simulink model "Vehicle14DOFSystemRack"  (R2024a)
settings: Solver=ode4  StartTime=0.0  StopTime=100  FixedStep=0.001  RelTol=1e-3
values from neighbouring files (symbols this model uses):
  EnvGrvty = 9.81    [Par.m]
  PlntBattChrgMax = 4.493    [Par.m]
  PlntBattNumCellSer = 96    [Par.m]
  PlntBattOpenCirctVolt = [3.17242 3.17242 3.17242 3.17242 3.17242 3.17242 3.17242;3.18272 3.18272 3.18272 3.18272 3.18272 3.18272 3.18272;3.19302 3.19302 3.19302 3.19302 3.19302 3.19302 3.19302;3.20331 3.20331 3.20331 3.20331 3.20331 3.20331 3.20331;3.21361 3.21361 3.21361 3.21361 3.21361 3.21361 3.21361;3.22391 3.22391 3.22391 3.22391 3.22391 3.22391 3.22391;3.23421 3.23421 3.23421 3.23421 3.23421 3.23421 3.23421;3.24451 ...(+5187 chars)    [Par.m]
  PlntBattSocInit = 0.6    [Par.m]
  PlntBattTempBpt = [-40 -30 -20 0 23 45 60]    [Par.m]
  PlntBattTempInitDegC = 25    [Par.m]
  PlntBattVoltSocBpt = [0 0.01 0.02 0.03 0.04 0.05 0.06 0.07 0.08 0.09 0.1 0.11 0.12 0.13 0.14 0.15 0.16 0.17 0.18 0.19 0.2 0.21 0.22 0.23 0.24 0.25 0.26 0.27 0.28 0.29 0.3 0.31 0.32 0.33 0.34 0.35 0.36 0.37 0.38 0.39 0.4 0.41 0.42 0.43 0.44 0.45 0.46 0.47 0.48 0.49 0.5 0.51 0.52 0.53 0.54 0.55 0.56 0.57 0.58 0.59 0.6 0.61 0.62 0.63 0.64 0.65 0.66 0.67 0.68 0.69 0.7 0.71 0.72 0.73 0.74 0.75 0.76 0.77 0.78 0.79 0.8 0.81  ...(+91 chars)    [Par.m]
  PlntDCDCVoltInit = 650    [Par.m]
  PlntDriveshftDamp = 100    [Par.m]
  PlntDriveshftStiff = 500    [Par.m]
  PlntEM1RotDamp = 0.001    [Par.m]
  PlntEM1RotInertia = 0.01    [Par.m]
  PlntEM2RotDamp = 0.001    [Par.m]
  PlntEM2RotInertia = 0.01    [Par.m]
  PlntEM3RotDamp = 0.001    [Par.m]
  PlntEM3RotInertia = 0.01    [Par.m]
  PlntEM4RotDamp = 0.001    [Par.m]
  PlntEM4RotInertia = 0.01    [Par.m]
  PlntEMWhlGearRatioFL = 11.04    [Par.m]
  PlntEMWhlGearRatioFR = 11.04    [Par.m]
  PlntEMWhlGearRatioRL = 11.04    [Par.m]
  PlntEMWhlGearRatioRR = 11.04    [Par.m]
  PlntSteerGearRatio = 52.025    [Par.m]
  PlntVehCGHgtAxl = 0.375    [Par.m]
  PlntVehDstCGFrntAxl = 1.61    [Par.m]
  PlntVehDstCGRearAxl = 1.39    [Par.m]
  PlntVehFrntUnsprgMass = 100    [Par.m]
  PlntVehInitLatPos = 0    [Par.m]
  PlntVehInitLatVel = 0    [Par.m]
  PlntVehInitLongPos = 0    [Par.m]
  PlntVehInitLongVel = 0    [Par.m]
  PlntVehInitPitchAng = 0    [Par.m]
  PlntVehInitPitchRate = 0    [Par.m]
  PlntVehInitRollAng = 0    [Par.m]
  PlntVehInitRollRate = 0    [Par.m]
  PlntVehInitVertPos = 0    [Par.m]
  PlntVehInitVertVel = 0    [Par.m]
  PlntVehInitYawAng = 0    [Par.m]
  PlntVehInitYawRate = 0    [Par.m]
  PlntVehMass = 2497    [Par.m]
  PlntVehPitchMomentInertia = 1922.7    [Par.m]
  PlntVehRearUnsprgMass = 100    [Par.m]
  PlntVehRollMomentInertia = 432.33333333333331    (= 432.333333333)    [Par.m]
  PlntVehTrckWdth = [1.685,1.685]    [Par.m]
  PlntVehYawMomentInertia = 2066    [Par.m]
  PlntWhlNumFrnt = 2    [Par.m]
  PlntWhlNumRear = 2    [Par.m]
  PlntWhlPrsFrnt = 220000    [Par.m]
  PlntWhlPrsRear = 220000    [Par.m]
libraries: autolibsharedcoupling x12, autolibsharedcommon x12, autolibutils x10, autolibmappedmotor x4, autolibcoupling x4, matrix_library x4, vehdynlibsteering x4, vehdynlibsuspension x2, vehdynlibtire x2, vehdynlibtirecommon x2, shared6dof x2, autolibdatasheetbattery x1
(part 6 of 7)

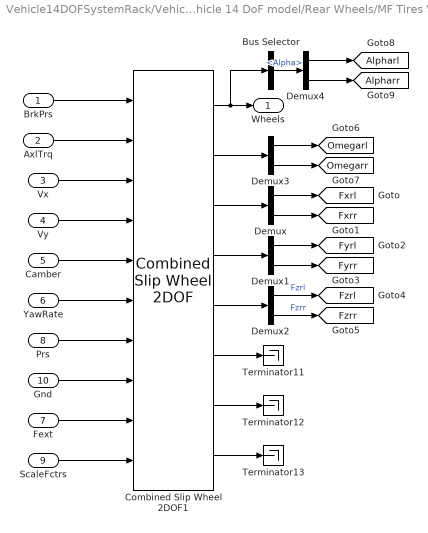
== system Vehicle14DOFSystemRack/Vehicle 14 DoF model/Vehicle 14 DoF model/Rear Wheels/MF Tires Vector ==
  BrkPrs : Inport
  AxlTrq : Inport  Port=2
  Vx : Inport  Port=3
  Vy : Inport  Port=4
  Camber : Inport  Port=5
  YawRate : Inport  Port=6
  Fext : Inport  Port=7
  Prs : Inport  Port=8  Unit=Pa
  ScaleFctrs : Inport  Port=9  Unit=1
  Gnd : Inport  Port=10
  Bus Selector : BusSelector  OutputSignals=Alpha
  Combined Slip Wheel 2DOF1 : vehdynlibtire/Combined Slip Wheel 2DOF  tireType=SUV 265/50R20  BrakeType=Disc  vertType=Magic Formula  plySteer=off  turnslip=on  mu_static=.3  mu_kinetic=.2  disk_abore=.05  Rm=.177  num_pads=2  drum_abore=0.0508  drum_a=0.123  drum_c=0.212  drum_r=0.15  drum_theta1=0  drum_theta2=126  brake_p_bpt=[1 11.4736842105263 21.9473684210526 32.4210526315789 42.8947368421053 53.3684210526316 63.8421052631579 74.3157894736842 84.7894736842105 95.2631578947368 105.736842105263 116.210526315789 126.684210526316 137.157894736842 147.631578947368 158.105263157895 168.578947368421 179.052631578947 189.526315789474 200]  brake_n_bpt=[0 52.6315789473684 105.263157894737 157.894736842105 210.526315789474 263.157894736842 315.789473684211 368.421052631579 421.052631578947 473.684210526316 526.315789473684 578.947368421053 631.578947368421 684.210526315789 736.842105263158 789.473684210526 842.105263157895 894.736842105263 947.368421052632 1000]  f_brake_t=[43.4900602404453 42.5056030554862 41.5350898940194 40.5780454442085 39.6340111501808 38.7025443887544 37.7832176914519 36.8756180088306 35.9793460143796 35.0940154454303 34.2192524787115 33.3546951383474 32.4999927342521 31.6548053290159 30.8188032315107 29.991666515561 29.1730845621415 28.362755623661 27.5603864089927 26.765691687993;498.991217495636 487.695866636631 476.560505099801 465.579679307235 454.748127933653 444.060772460445 433.51270824929 423.099196101319 412.81565427025 402.657650900201 392.620896861006 382.701238955775 372.894653477208 363.197240090814 353.605216024701 344.114910546964 334.722759712992 325.425301366216 316.219170376863 307.10109410434;954.492374750826 932.886130217776 911.585920305583 890.581313170261 869.862244717126 849.419000532136 829.242198807128 809.322774193808 789.651962526121 770.221286354971 751.0225412433 732.047782773203 713.289314220164 694.739674852612 676.391628817892 658.238154578366 640.272434863842 622.48784710877 604.877954344734 587.436496520688;1409.99353200602 1378.07639379892 1346.61133551136 1315.58294703329 1284.9763615006 1254.77722860383 1224.97168936497 1195.5463522863 1166.48827078199 1137.78492180974 1109.42418562559 1081.39432659063 1053.68397496312 1026.28210961441 999.178041611083 972.361398609768 945.822110014692 919.550392851325 893.536738312604 867.771898937035;1865.49468926121 1823.26665738007 1781.63675071715 1740.58458089631 1700.09047828407 1660.13545667552 1620.7011799228 1581.76993037878 1543.32457903786 1505.34855726451 1467.82583000789 1430.74087040806 1394.07863570608 1357.82454437621 1321.96445440427 1286.48464264117 1251.37178516554 1216.61293859388 1182.19552228048 1148.10730135338;2320.9958465164 2268.45692096121 2216.66216592293 2165.58621475934 2115.20459506754 2065.49368474721 2016.43067048064 1967.99350847127 1920.16088729373 1872.91219271928 1826.22747439018 1780.08741422549 1734.47329644903 1689.36697913801 1644.75086719747 1600.60788667257 1556.92146031639 1513.67548433643 1470.85430624835 1428.44270376973;2776.49700377159 2713.64718454235 2651.68758112871 2590.58784862237 2530.31871185102 2470.8519128189 2412.16016103848 2354.21708656376 2296.9971955496 2240.47582817405 2184.62911877248 2129.43395804292 2074.86795719199 2020.9094138998 1967.53727999066 1914.73113070398 1862.47113546724 1810.73803007899 1759.51309021622 1708.77810618608;3231.99816102678 3158.8374481235 3086.71299633449 3015.58948248539 2945.43282863449 2876.21014089059 2807.88965159632 2740.44066465625 2673.83350380547 2608.03946362882 2543.03076315477 2478.78050186034 2415.26261793494 2352.4518486616 2290.32369278385 2228.85437473538 2168.02081061809 2107.80057582154 2048.17187418409 1989.11350860242;3687.49931828197 3604.02771170464 3521.73841154027 3440.59111634842 3360.54694541796 3281.56836896228 3203.61914215416 3126.66424274874 3050.66981206134 2975.60309908359 2901.43240753707 2828.12704567777 2755.6572786779 2683.9942834234 2613.11010557704 2542.97761876678 2473.57048576894 2404.8631215641 2336.83065815196 2269.44891101877;4143.00047553716 4049.21797528579 3956.76382674606 3865.59275021144 3775.66106220143 3686.92659703397 3599.34863271199 3512.88782084123 3427.50612031721 3343.16673453836 3259.83405191936 3177.4735894952 3096.05193942085 3015.5367181852 2935.89651837023 2857.10086279818 2779.12016091979 2701.92566730665 2625.48944211983 2549.78431343512;4598.50163279235 4494.40823886693 4391.78924195184 4290.59438407447 4190.77517898491 4092.28482510566 3995.07812326983 3899.11139893372 3804.34242857308 3710.73036999313 3618.23569630166 3526.82013331263 3436.44660016381 3347.079152947 3258.68293116342 3171.22410682959 3084.66983607064 2998.98821304921 2914.1482260877 2830.11971585147;5054.00279004754 4939.59850244808 4826.81465715762 4715.59601793749 4605.88929576838 4497.64305317735 4390.80761382767 4285.3349770262 4181.17873682896 4078.2940054479 3976.63734068395 3876.16667713006 3776.84126090677 3678.62158770879 3581.46934395661 3485.34735086099 ...(+2764 chars)]  tireParamSet=vdynPassCar.mat  PRESMAX=1000000  PRESMIN=10000  FZMAX=12400  FZMIN=100  VXLOW=0.1  KPUMAX=1.5  KPUMIN=-1.5  ALPMAX=1.5  ALPMIN=-1.5  CAMMAX=0.17453  CAMMIN=-0.17453  LONGVL=16.7  FxRelFreqLwrLim=200*pi  FyRelFreqLwrLim=200*pi  MyRelFreqLwrLim=100*pi  omegao=20/0.3869  br=1e-3  UNLOADED_RADIUS=0.3869  NOMPRES=269000  FNOMIN=6200  WIDTH=0.265  RIM_RADIUS=0.254  MASS=16.15  IYY=2.081  GRAVITY=-9.81  zo=0  zdoto=0  BREFF=8.25094594147963  DREFF=0.260468730454265  FREFF=0.0735298544471851  Q_RE0=1.00866439868088  Q_V1=0.000760413786224011  Q_V2=0.0463384792019201  Q_FZ1=0  Q_FZ2=15.6870832810226  Q_FZ3=0  Q_FCX=0.138643970247602  Q_FCY=0.10843499565426  Q_FCY2=-0.465763352339538  PFZ1=0.69958166705601  VERTICAL_STIFFNESS=207885.061134007  VERTICAL_DAMPING=500  BOTTOM_OFFST=.01  BOTTOM_STIFF=2e6  LONGITUDINAL_STIFFNESS=388714.175879854  LATERAL_STIFFNESS=157087.404633332  PCFX1=0.18539229191199  PCFX2=0  PCFX3=0  PCFY1=0.163183345037677  PCFY2=0  PCFY3=0.249094918231954  Q_RA1=0.675942571700787  Q_RA2=0.73800463546164  Q_RB1=1.04487486456705  Q_RB2=-1.191763806629  PCX1=1.58523057950359  PDX1=1.0239116238178  PDX2=-0.0842405110022724  PDX3=0  PEX1=0.110312777158455  PEX2=0.313468516038146  PEX3=0  PEX4=0.0016060905760045  PKX1=21.3872544684023  PKX2=14.0006541873175  PKX3=-0.405326109653452  PHX1=0.000212599305364818  PHX2=0.00115950515263055  PVX1=1.59236164471432e-05  PVX2=0.000104321112127671  PPX1=-0.349461321276586  PPX2=0.387840040616429  PPX3=-0.0969947336569324  PPX4=0.0632271859795801  RBX1=12.7633329850276  RBX2=9.5787123658471  RBX3=0  RCX1=1.02796280922059  REX1=-0.45202516851367  REX2=-0.47304886171176  RHX1=0.000233272373115809  QSX1=-0.00788307788961443  QSX2=0.954629515459396  QSX3=0.0155855777667025  QSX4=0.125904607142414  QSX5=1.01110069703963  QSX6=20.1938577118433  QSX7=0.310818120717083  QSX8=-0.0430823751139655  QSX9=0.636494404888216  QSX10=0.142438060591663  QSX11=0.346766530036373  QSX12=0  QSX13=0  QSX14=0  PPMX1=0  PCY1=1.34299950037631  PDY1=0.878267729082195  PDY2=-0.0644597923147385  PDY3=0  PEY1=-0.809776534470972  PEY2=-0.600180598867198  PEY3=0.0991732552633487  PEY4=-6.5577974035573  PEY5=0  PKY1=-15.5714726518315  PKY2=1.73126522291751  PKY3=0.365349873517229  PKY4=1.98176755955416  PKY5=0  PKY6=-0.884005199550313  PKY7=-0.237259727611847  PHY1=-0.00183370557235628  PHY2=0.00346401302716671  PVY1=-0.00675427560163264  PVY2=0.036379218103843  PVY3=-0.163543984089166  PVY4=-0.491003349625726  PPY1=-0.62059646553185  PPY2=-0.0647824842338686  PPY3=-0.164648843290686  PPY4=0.283193909060098  PPY5=0  RBY1=10.7588809173639  RBY2=7.70420065295029  RBY3=3.40283755070691e-06  RBY4=0  RCY1=1.06691874059059  REY1=0.308244924574305  REY2=7.48775032604508e-06  RHY1=0.0118479204960415  RHY2=7.63650177161071e-06  RVY1=0.0560024425050078  RVY2=7.48487127056197e-06  RVY3=0  RVY4=98.4047026517149  RVY5=2.02759273900054  RVY6=15.7623064923347  QSY1=0.00699077564863536  QSY2=0  QSY3=0.00153535478298811  QSY4=8.55710322455322e-05  QSY5=0  QSY6=0  QSY7=0.89443879773793  QSY8=-0.403227641260894  QBZ1=11.666656027484  QBZ2=-1.30355438574485  QBZ3=0  QBZ4=0.177918305399071  QBZ5=-0.162481135068033  QBZ6=0  QBZ9=30.1445534682089  QBZ10=0  QCZ1=1.29026978207574  QDZ1=0.0886972644991399  QDZ2=-0.0058634820161856  QDZ3=0.3805597481383  QDZ4=0  QDZ6=0.00160914918118959  QDZ7=-0.00211036330862154  QDZ8=-0.13921904912557  QDZ9=0.00816585550028243  QDZ10=0  QDZ11=0  QEZ1=-2.19802254534746  QEZ2=1.01850535789165  QEZ3=0  QEZ4=0.278379679112054  QEZ5=-0.548414722765386  QHZ1=0.00148361198869669  QHZ2=0.00202017567585904  QHZ3=0.240316641332066  QHZ4=-0.210114035738085  PPZ1=-0.443927982388615  PPZ2=0  SSZ1=0.00914999585397887  SSZ2=0.0389830656052735  SSZ3=0  SSZ4=0  PDXP1=0.396718274678791  PDXP2=0  PDXP3=0  PKYP1=1.00587060633573  PDYP1=0.40483048923438  PDYP2=0  PDYP3=0  PDYP4=0  PHYP1=0.992731942067188  PHYP2=0.150352945499914  PHYP3=0  PHYP4=-3.98988682633674  PECP1=0.502379254513503  PECP2=0  QDTP1=10.0178654287947  QCRP1=0.200627747200702  QCRP2=0.0995735881599772  QBRP1=0.0997107127960717  QDRP1=1.01432910167423  QDRP2=0  aMode=2
  Demux{,1..4} (5 alike) : Demux  Outputs=2
  Terminator11 : Terminator
  Terminator12 : Terminator
  Terminator13 : Terminator
  Wheels : Outport  VectorParamsAs1DForOutWhenUnconnected=off
  tag scope: Alpharl=global, Alpharr=global, Fxrl=global, Fxrr=global, Fyrl=global, Fyrr=global, Fzrl=global, Fzrr=global, Omegarl=global, Omegarr=global
  wires:
  Vy/1 -> Combined Slip Wheel 2DOF1/4
  Combined Slip Wheel 2DOF1/8 -> Terminator13/1
  Combined Slip Wheel 2DOF1/7 -> Terminator12/1
  Combined Slip Wheel 2DOF1/6 -> Terminator11/1
  Fext/1 -> Combined Slip Wheel 2DOF1/9
  Gnd/1 -> Combined Slip Wheel 2DOF1/8
  Prs/1 -> Combined Slip Wheel 2DOF1/7
  YawRate/1 -> Combined Slip Wheel 2DOF1/6
  Camber/1 -> Combined Slip Wheel 2DOF1/5
  Vx/1 -> Combined Slip Wheel 2DOF1/3
  AxlTrq/1 -> Combined Slip Wheel 2DOF1/2
  BrkPrs/1 -> Combined Slip Wheel 2DOF1/1
  ScaleFctrs/1 -> Combined Slip Wheel 2DOF1/10
  Demux3/2 -> [Omegarr]
  Demux3/1 -> [Omegarl]
  Demux1/2 -> [Fyrr]
  Demux1/1 -> [Fyrl]
  Combined Slip Wheel 2DOF1/2 -> Demux3/1
  Combined Slip Wheel 2DOF1/4 -> Demux1/1
  Combined Slip Wheel 2DOF1/5 -> Demux2/1
  Demux2/2 -> [Fzrr]  "Fzrr"
  Combined Slip Wheel 2DOF1/3 -> Demux/1
  Demux2/1 -> [Fzrl]  "Fzrl"
  Demux/2 -> [Fxrr]
  Demux/1 -> [Fxrl]
  Combined Slip Wheel 2DOF1/1 -> Bus Selector/1, Wheels/1
  Demux4/1 -> [Alpharl]
  Bus Selector/1 -> Demux4/1  "<Alpha>"
  Demux4/2 -> [Alpharr]

== system Vehicle14DOFSystemRack/Vehicle 14 DoF model/Vehicle 14 DoF model/Rear Wheels/Rear Friction ==
  u : Inport
  Selector1 : Selector  InputPortWidth=4  IndexOptions=Index vector (dialog)  Indices=[3 4]  OutputSizes=1
  y : Outport
  wires:
  Selector1/1 -> y/1
  u/1 -> Selector1/1

== system Vehicle14DOFSystemRack/Vehicle 14 DoF model/Vehicle 14 DoF model/Rear Wheels/Rear Ground ==
  u : Inport
  Selector1 : Selector  InputPortWidth=4  IndexOptions=Index vector (dialog)  Indices=[3 4]  OutputSizes=1
  y : Outport
  wires:
  u/1 -> Selector1/1
  Selector1/1 -> y/1

== system Vehicle14DOFSystemRack/Vehicle 14 DoF model/Vehicle 14 DoF model/Rear Wheels/Subsystem ==
  lamda_mu_x : Inport
  lamda_mu_y : Inport  Port=2
  Rear Pressure : vehdynlibtirecommon/Constant  const=PlntWhlPrsRear  numWheels=PlntWhlNumRear
  scale factors with friction : Subsystem  mask{numWheels=PlntWhlNumRear}
      mask prompts: numWheels "Number of wheels"
  Prs : Outport
  ScaleFctrs : Outport  Port=2
  wires:
  lamda_mu_y/1 -> scale factors with friction/2(lamda_mu_y)
  scale factors with friction/1(lambdas) -> ScaleFctrs/1
  lamda_mu_x/1 -> scale factors with friction/1(lamda_mu_x)
  Rear Pressure/1 -> Prs/1

== system Vehicle14DOFSystemRack/Vehicle 14 DoF model/Vehicle 14 DoF model/Transfer Case/DriveshftTrq Routing ==
  TrnsfrCaseFrntTrq : Inport
  DriveshftTrq : Inport  Port=2
  "TrnsfrCaseRearTrq " : Inport  Port=3
  Constant : Constant  Value=0  SampleTime=-1
  FrntDiffrntlTrq : Outport
  TrnsfrCaseTrq : Outport  Port=2
  RearDiffrntlTrq : Outport  Port=3
  wires:
  DriveshftTrq/1 -> FrntDiffrntlTrq/1, RearDiffrntlTrq/1
  Constant/1 -> TrnsfrCaseTrq/1

== system Vehicle14DOFSystemRack/Vehicle 14 DoF model/Vehicle 14 DoF model/Transfer Case/Subsystem ==
  TrqSplitRatio : Inport
  SpdLock : Inport  Port=2
  FrntDiffrntlSpd : Inport  Port=3
  DriveshftTrq : Inport  Port=4
  RearDiffrntlSpd : Inport  Port=5
  Constant : Constant  Value=0  SampleTime=-1
  Constant1 : Constant  Value=0  SampleTime=-1
  Constant2 : Constant  Value=0  SampleTime=-1
  DriveshftSpd : Outport
  FrntDiffrntlTrq : Outport  Port=2
  RearDiffrntlTrq : Outport  Port=3
  wires:
  Constant2/1 -> RearDiffrntlTrq/1
  Constant1/1 -> FrntDiffrntlTrq/1
  Constant/1 -> DriveshftSpd/1

== system Vehicle14DOFSystemRack/Vehicle 14 DoF model/Vehicle 14 DoF model/Transmission/BEV4 ==
  EMTrq : Inport
  DriveshftSpd : Inport  Port=2
  Bus Creator : BusCreator  Inputs=4
  Bus Creator1 : BusCreator  Inputs=4
  Bus Selector : BusSelector  OutputSignals=FrntDriveshftSpd.DriveshftSpd1
  Bus Selector1 : BusSelector  OutputSignals=FrntDriveshftSpd.DriveshftSpd2
  Bus Selector2 : BusSelector  OutputSignals=RearDriveshftSpd.DriveshftSpd3
  Bus Selector3 : BusSelector  OutputSignals=RearDriveshftSpd.DriveshftSpd4
  Bus Selector4 : BusSelector  OutputSignals=EMTrq1
  Bus Selector5 : BusSelector  OutputSignals=EMTrq2
  Bus Selector6 : BusSelector  OutputSignals=EMTrq3
  Bus Selector7 : BusSelector  OutputSignals=EMTrq4
  Driveshaft Compliance{,1..3} (4 alike) : autolibsharedcoupling/Torsional Compliance  port_config=Simulink  extInfo=off  k=PlntDriveshftStiff  b=PlntDriveshftDamp  theta_o=PlntDriveshftInitDeflect  domega_o=PlntDriveshftInitVel  omega_c=PlntDriveshftDampCutoffFreq  blkID=0  aMode=1
  Rotational Inertia : autolibsharedcoupling/Rotational Inertia  port_config=Simulink  extInfo=off  externJ=off  J=PlntEM1RotInertia  b=PlntEM1RotDamp  omega_o=PlntEM1RotInitSpd  blkID=0  aMode=1
      settings: LibrarySourceBlock=autolibcoupling/Rotational Inertia
  Rotational Inertia1 : autolibsharedcoupling/Rotational Inertia  port_config=Simulink  extInfo=off  externJ=off  J=PlntEM2RotInertia  b=PlntEM2RotDamp  omega_o=PlntEM2RotInitSpd  blkID=0  aMode=1
      settings: LibrarySourceBlock=autolibcoupling/Rotational Inertia
  Rotational Inertia2 : autolibsharedcoupling/Rotational Inertia  port_config=Simulink  extInfo=off  externJ=off  J=PlntEM3RotInertia  b=PlntEM3RotDamp  omega_o=PlntEM3RotInitSpd  blkID=0  aMode=1
      settings: LibrarySourceBlock=autolibcoupling/Rotational Inertia
  Rotational Inertia3 : autolibsharedcoupling/Rotational Inertia  port_config=Simulink  extInfo=off  externJ=off  J=PlntEM4RotInertia  b=PlntEM4RotDamp  omega_o=PlntEM4RotInitSpd  blkID=0  aMode=1
      settings: LibrarySourceBlock=autolibcoupling/Rotational Inertia
  EMSpd : Outport  VectorParamsAs1DForOutWhenUnconnected=off  BusOutputAsStruct=on
  DriveshftTrq : Outport  Port=2  VectorParamsAs1DForOutWhenUnconnected=off
  wires:
  Bus Selector2/1 -> Driveshaft Compliance2/2  "<DriveshftSpd3>"
  Rotational Inertia1/1 -> Bus Creator1/2, Driveshaft Compliance1/1  "EMSpd2"
  Bus Creator/1 -> DriveshftTrq/1
  Bus Selector4/1 -> Rotational Inertia/1  "<EMTrq1>"
  EMTrq/1 -> Bus Selector4/1, Bus Selector5/1, Bus Selector7/1, Bus Selector6/1
  Bus Selector3/1 -> Driveshaft Compliance3/2  "<DriveshftSpd4>"
  Rotational Inertia/1 -> Bus Creator1/1, Driveshaft Compliance/1  "EMSpd1"
  Bus Selector/1 -> Driveshaft Compliance/2  "<DriveshftSpd1>"
  Bus Selector7/1 -> Rotational Inertia3/1  "<EMTrq4>"
  Driveshaft Compliance3/1 -> Rotational Inertia3/2
  Driveshaft Compliance/1 -> Rotational Inertia/2
  Bus Selector5/1 -> Rotational Inertia1/1  "<EMTrq2>"
  Driveshaft Compliance1/1 -> Rotational Inertia1/2
  DriveshftSpd/1 -> Bus Selector/1, Bus Selector1/1, Bus Selector3/1, Bus Selector2/1
  Driveshaft Compliance3/2 -> Bus Creator/4  "DriveshftTrq4"
  Bus Creator1/1 -> EMSpd/1
  Driveshaft Compliance2/1 -> Rotational Inertia2/2
  Rotational Inertia2/1 -> Bus Creator1/3, Driveshaft Compliance2/1  "EMSpd3"
  Bus Selector1/1 -> Driveshaft Compliance1/2  "<DriveshftSpd2>"
  Rotational Inertia3/1 -> Bus Creator1/4, Driveshaft Compliance3/1  "EMSpd4"
  Bus Selector6/1 -> Rotational Inertia2/1  "<EMTrq3>"
  Driveshaft Compliance2/2 -> Bus Creator/3  "DriveshftTrq3"
  Driveshaft Compliance1/2 -> Bus Creator/2  "DriveshftTrq2"
  Driveshaft Compliance/2 -> Bus Creator/1  "DriveshftTrq1"

== system Vehicle14DOFSystemRack/Vehicle 14 DoF model/Vehicle 14 DoF model/Vehicle Body/Subsystem ==
  Veh : Inport
  Bus Creator : BusCreator  Inputs=2
  Bus Selector : BusSelector  OutputSignals=BdyFrm.Cg.Acc.ax,BdyFrm.Cg.Acc.ay,BdyFrm.Cg.Acc.az  OutputAsBus=on
  Bus Selector1 : BusSelector  OutputSignals=BdyFrm.Cg.AngVel.p,BdyFrm.Cg.AngVel.q,BdyFrm.Cg.AngVel.r  OutputAsBus=on
  Bus Selector2 : BusSelector  OutputSignals=BdyFrm.Cg.AngAcc.pdot,BdyFrm.Cg.AngAcc.qdot,BdyFrm.Cg.AngAcc.rdot  OutputAsBus=on
  Bus to Vector : BusToVector
  Bus to Vector1 : BusToVector
  Bus to Vector2 : BusToVector
  Constant : Constant  Value=[0,0,0]
  Constant1 : Constant  Value=[0,0,9.81]
  Three-axis Inertial Measurement Unit : vehdynlibsens/Three-axis Inertial Measurement Unit  units=Metric (MKS)  imu=[0 0 0]  i_Ts=0  dtype_a=off  w_a=190  z_a=0.707  a_sf_cc=[1 0 0; 0 1 0; 0 0 1]  a_bias=[0 0 0]  a_sat="[-inf  -inf  -inf  inf inf inf]"  dtype_g=off  w_g=190  z_g=0.707  g_sf_cc=[1 0 0; 0 1 0; 0 0 1]  g_bias=[0 0 0]  g_sens=[0 0 0]  g_sat="[-inf  -inf  -inf  inf inf inf]"  i_rand=on  i_seeds=[23093 23094 23095 23096 23097 23098]  i_pow=[0.001 0.001 0.001 0.0001 0.0001 0.0001]  aMode=2
  Unit Conversion : UnitConversion
  IMU : Outport
  wires:
  Three-axis Inertial Measurement Unit/2 -> Bus Creator/2  "Omega"
  Veh/1 -> Bus Selector2/1, Bus Selector1/1, Bus Selector/1
  Constant1/1 -> Three-axis Inertial Measurement Unit/5
  Bus to Vector1/1 -> Three-axis Inertial Measurement Unit/2
  Bus to Vector/1 -> Unit Conversion/1
  Bus Selector1/1 -> Bus to Vector1/1
  Constant/1 -> Three-axis Inertial Measurement Unit/4
  Three-axis Inertial Measurement Unit/1 -> Bus Creator/1  "Ameans"
  Bus Selector2/1 -> Bus to Vector2/1
  Unit Conversion/1 -> Three-axis Inertial Measurement Unit/1
  Bus to Vector2/1 -> Three-axis Inertial Measurement Unit/3
  Bus Selector/1 -> Bus to Vector/1
  Bus Creator/1 -> IMU/1

== system Vehicle14DOFSystemRack/Vehicle 14 DoF model/Vehicle 14 DoF model/Vehicle Body/Vehicle 6DOF ==
  Suspension : Inport
  Constant{1..4} (4 alike) : Constant  Value=[0;0;0]  SampleTime=-1
  Suspension to Chasiss Transforms : Subsystem
  Terminator{,1..5} (6 alike) : Terminator
  Vehicle Body 6DOF : vehdynlibeom/Vehicle Body 6DOF  extPos=on  extVel=on  extEuler=on  extRotRate=on  htchFMode=on  htchMMode=on  m=PlntVehMass  a=PlntVehDstCGFrntAxl  b=PlntVehDstCGRearAxl  d=0  h=PlntVehCGHgtAxl  dh=PlntVehHtchDst  hl=0  hh=PlntVehHtchHgtAxl  Xe_o=[PlntVehInitLongPos, PlntVehInitLatPos, PlntVehInitVertPos]  xbdot_o=[PlntVehInitLongVel+20, PlntVehInitLatVel, PlntVehInitVertVel]  eul_o=[PlntVehInitRollAng, PlntVehInitPitchAng, PlntVehInitYawAng]  p_o=[PlntVehInitRollRate, PlntVehInitPitchRate, PlntVehInitYawRate]  Iveh=[PlntVehRollMomentInertia 0 0; 0 PlntVehPitchMomentInertia 0; 0 0 PlntVehYawMomentInertia]  w=PlntVehTrckWdth  z1m=0  z1R=[-.25,.125,.15]  z1I=[1.4,-.2,.1;-.2,1.4,.1;.1,.1,2.25].*0  z2m=0  z2R=[1.4,0,.8]  z2I=[1.4,-.2,.1;-.2,1.4,.1;.1,.1,2.25].*0  z3m=0  z3R=[.75,-.5,.4]  z3I=[5,-.1,-2;-2,9,.1;-.1,.1,6].*0  z4m=0  z4R=[.75,.5,.4]  z4I=[5,-.1,-2;-2,9,.1;-.1,.1,6].*0  z5m=0  z5R=[1.25,-.5,.4]  z5I=[5,-.1,-2;-2,9,.1;-.1,.1,6].*0  z6m=0  z6R=[1.25,-.5,.4]  z6I=[5,-.1,-2;-2,9,.1;-.1,.1,6].*0  z7m=0  z7R=[2,0,.25]  z7I=[1.4,-.2,.1;-.2,1.4,.1;.1,.1,2.25].*0  Af=PlntVehAeroFrntArea  Cd=PlntVehAeroDragCff  Cl=PlntVehAeroLiftCff  Cpm=PlntVehAeroPitchCff  beta_w=[0 0.01:0.01:0.3]  Cs=[0 0.01:0.01:0.3]  Cym=[0 1e-6:0.01:0.3]  Pabs=EnvAbsPrs  extTamb=off  Tair=EnvAirTemp  g=EnvGrvty  xdot_tol=.1  longOff=0  latOff=0  vertOff=0.0112  wrapAng=off  aMode=2
  Veh : Outport
  wires:
  Vehicle Body 6DOF/2 -> Terminator/1
  Suspension to Chasiss Transforms/1(FsB) -> Vehicle Body 6DOF/1
  Vehicle Body 6DOF/1 -> Veh/1, Suspension to Chasiss Transforms/1(VehFdbk)  "VehFdbk"
  Suspension/1 -> Suspension to Chasiss Transforms/2(Suspension)
  Suspension to Chasiss Transforms/2(MsB) -> Vehicle Body 6DOF/2
  Suspension to Chasiss Transforms/3(Fext) -> Vehicle Body 6DOF/3
  Vehicle Body 6DOF/7 -> Terminator5/1
  Vehicle Body 6DOF/6 -> Terminator4/1
  Vehicle Body 6DOF/4 -> Terminator2/1
  Vehicle Body 6DOF/3 -> Terminator1/1
  Vehicle Body 6DOF/5 -> Terminator3/1
  Constant2/1 -> Vehicle Body 6DOF/5
  Constant1/1 -> Vehicle Body 6DOF/4
  Constant3/1 -> Vehicle Body 6DOF/6
  Constant4/1 -> Vehicle Body 6DOF/7

== system Vehicle14DOFSystemRack/Vehicle 14 DoF model/Vehicle 14 DoF model/Front Suspension/Kinematics and Compliance Independent Suspension/Calculate dynamic track width from lateral wheel center displacement change ==
  dWhlY : Inport
  dWhlZ : Inport  Port=2
  Front Track Calculation : Subsystem
  Gain : Gain  Gain=-1
  Rear Track Calculation : Subsystem
  Sign : Signum  ZeroCross=off
  Vector Concatenate : Concatenate
  w : Outport
  wires:
  Gain/1 -> Sign/1
  Sign/1 -> Front Track Calculation/2(sign), Rear Track Calculation/2(sign)
  Rear Track Calculation/1(w_rear) -> Vector Concatenate/2
  Front Track Calculation/1(w_front) -> Vector Concatenate/1
  Vector Concatenate/1 -> w/1
  dWhlY/1 -> Front Track Calculation/1(dWhlY), Rear Track Calculation/1(dWhlY)
  dWhlZ/1 -> Gain/1

== system Vehicle14DOFSystemRack/Vehicle 14 DoF model/Vehicle 14 DoF model/Front Suspension/Kinematics and Compliance Independent Suspension/Steer Rate Adapter ==
  Veh : Inport
  Add : Sum
  Bus Selector3 : BusSelector  OutputSignals=BdyFrm.Cg.AngVel.r
  Constant : Constant  Value=zeros(1,4)  SampleTime=-1
  Matrix Concatenate : Concatenate  NumInputs=3  Mode=Multidimensional array
  Matrix Concatenate1 : Concatenate  NumInputs=3  Mode=Multidimensional array
  Reshape2 : Reshape  OutputDimensionality=Row vector (2-D)
  Reshape3 : Reshape  OutputDimensionality=Row vector (2-D)
  Reshape4 : Reshape  OutputDimensionality=Row vector (2-D)
  Selector3 : Selector  InputPortWidth=1  IndexOptions=Index vector (dialog)  Indices=[1 1 1 1]  OutputSizes=1
  SteerRates : Constant  Value=zeros(1,4)  SampleTime=-1
  AngVel : Outport  VectorParamsAs1DForOutWhenUnconnected=off
  wires:
  Add/1 -> AngVel/1  "AngVel"
  Veh/1 -> Bus Selector3/1
  Matrix Concatenate1/1 -> Add/1
  Reshape3/1 -> Matrix Concatenate/1, Matrix Concatenate/2
  Reshape4/1 -> Matrix Concatenate/3
  SteerRates/1 -> Reshape2/1
  Matrix Concatenate/1 -> Add/2
  Bus Selector3/1 -> Selector3/1  "<r>"
  Selector3/1 -> Reshape4/1
  Constant/1 -> Reshape3/1
  Reshape2/1 -> Matrix Concatenate1/2, Matrix Concatenate1/3, Matrix Concatenate1/1

== system Vehicle14DOFSystemRack/Vehicle 14 DoF model/Vehicle 14 DoF model/Front Suspension/Kinematics and Compliance Independent Suspension/Steering Adapter ==
  Steer : Inport
  Reshape1 : Reshape  OutputDimensionality=Row vector (2-D)
  Selector : Selector  IndexOptions=Index vector (dialog)  Indices=[1 2]  OutputSizes=1
  StrgAng : Outport  VectorParamsAs1DForOutWhenUnconnected=off
  wires:
  Selector/1 -> Reshape1/1
  Steer/1 -> Selector/1
  Reshape1/1 -> StrgAng/1

== system Vehicle14DOFSystemRack/Vehicle 14 DoF model/Vehicle 14 DoF model/Front Suspension/Kinematics and Compliance Independent Suspension/Vehicle Adapter ==
  Veh : Inport
  Bus Creator3 : BusCreator  Inputs=2
  Bus Selector1 : BusSelector  OutputSignals=InertFrm.FrntAxl.Lft.Disp.X,InertFrm.FrntAxl.Lft.Disp.Y,InertFrm.FrntAxl.Lft.Disp.Z,InertFrm.FrntAxl.Rght.Disp.X,InertFrm.FrntAxl.Rght.Disp.Y,InertFrm.FrntAxl.Rght.Disp.Z,InertFrm.RearAxl.Lft.Disp.X,InertFrm.RearAxl.Lft.Disp.Y,InertFrm.RearAxl.Lft.Disp.Z,InertFrm.RearAxl.Rght.Disp.X,InertFrm.RearAxl.Rght.Disp.Y,InertFrm.RearAxl.Rght.Disp.Z
  Bus Selector2 : BusSelector  OutputSignals=BdyFrm.FrntAxl.Lft.Vel.xdot,BdyFrm.FrntAxl.Lft.Vel.ydot,BdyFrm.FrntAxl.Lft.Vel.zdot,BdyFrm.FrntAxl.Rght.Vel.xdot,BdyFrm.FrntAxl.Rght.Vel.ydot,BdyFrm.FrntAxl.Rght.Vel.zdot,BdyFrm.RearAxl.Lft.Vel.xdot,BdyFrm.RearAxl.Lft.Vel.ydot,BdyFrm.RearAxl.Lft.Vel.zdot,BdyFrm.RearAxl.Rght.Vel.xdot,BdyFrm.RearAxl.Rght.Vel.ydot,BdyFrm.RearAxl.Rght.Vel.zdot
  Bus Selector3 : BusSelector  OutputSignals=InertFrm.FrntAxl.Lft.Vel.Xdot,InertFrm.FrntAxl.Lft.Vel.Ydot,InertFrm.FrntAxl.Lft.Vel.Zdot,InertFrm.FrntAxl.Rght.Vel.Xdot,InertFrm.FrntAxl.Rght.Vel.Ydot,InertFrm.FrntAxl.Rght.Vel.Zdot,InertFrm.RearAxl.Lft.Vel.Xdot,InertFrm.RearAxl.Lft.Vel.Ydot,InertFrm.RearAxl.Lft.Vel.Zdot,InertFrm.RearAxl.Rght.Vel.Xdot,InertFrm.RearAxl.Rght.Vel.Ydot,InertFrm.RearAxl.Rght.Vel.Zdot
  Inertial Frame CG to Axle Offset : Constant  Value=[zeros(2,4);PlntVehCGHgtAxl*ones(1,4)]  SampleTime=-1
  Mux1 : Mux  Inputs=12
  Mux2 : Mux  Inputs=12
  Mux3 : Mux  Inputs=12
  Reshape : Reshape  OutputDimensionality=Customize  OutputDimensions=[3,4]
  Reshape1 : Reshape  OutputDimensionality=Customize  OutputDimensions=[3,4]
  Reshape2 : Reshape  OutputDimensionality=Customize  OutputDimensions=[3,4]
  Sum : Sum  Inputs=|+-
  VehSusp : Outport  VectorParamsAs1DForOutWhenUnconnected=off
  VehVbody : Outport  Port=2  VectorParamsAs1DForOutWhenUnconnected=off
  wires:
  Reshape1/1 -> Bus Creator3/2  "V"
  Bus Selector3/1 -> Mux3/1  "<Xdot>"
  Bus Selector3/2 -> Mux3/2  "<Ydot>"
  Bus Selector3/3 -> Mux3/3  "<Zdot>"
  Bus Selector3/4 -> Mux3/4  "<Xdot>"
  Bus Selector3/5 -> Mux3/5  "<Ydot>"
  Bus Selector3/6 -> Mux3/6  "<Zdot>"
  Bus Selector3/7 -> Mux3/7  "<Xdot>"
  Bus Selector3/8 -> Mux3/8  "<Ydot>"
  Bus Selector3/9 -> Mux3/9  "<Zdot>"
  Bus Selector3/10 -> Mux3/10  "<Xdot>"
  Bus Selector3/11 -> Mux3/11  "<Ydot>"
  Bus Selector3/12 -> Mux3/12  "<Zdot>"
  Mux3/1 -> Reshape1/1
  Sum/1 -> Bus Creator3/1  "P"
  Inertial Frame CG to Axle Offset/1 -> Sum/2
  Mux2/1 -> Reshape/1
  Mux1/1 -> Reshape2/1
  Bus Selector2/12 -> Mux1/12  "<zdot>"
  Bus Selector2/11 -> Mux1/11  "<ydot>"
  Bus Selector2/10 -> Mux1/10  "<xdot>"
  Bus Selector2/9 -> Mux1/9  "<zdot>"
  Bus Selector2/8 -> Mux1/8  "<ydot>"
  Bus Selector2/7 -> Mux1/7  "<xdot>"
  Bus Selector2/6 -> Mux1/6  "<zdot>"
  Bus Selector2/5 -> Mux1/5  "<ydot>"
  Bus Selector2/4 -> Mux1/4  "<xdot>"
  Bus Selector2/3 -> Mux1/3  "<zdot>"
  Bus Selector2/2 -> Mux1/2  "<ydot>"
  Bus Selector2/1 -> Mux1/1  "<xdot>"
  Bus Selector1/12 -> Mux2/12  "<Z>"
  Bus Selector1/11 -> Mux2/11  "<Y>"
  Bus Selector1/10 -> Mux2/10  "<X>"
  Bus Selector1/9 -> Mux2/9  "<Z>"
  Bus Selector1/8 -> Mux2/8  "<Y>"
  Bus Selector1/7 -> Mux2/7  "<X>"
  Bus Selector1/6 -> Mux2/6  "<Z>"
  Bus Selector1/5 -> Mux2/5  "<Y>"
  Bus Selector1/4 -> Mux2/4  "<X>"
  Bus Selector1/3 -> Mux2/3  "<Z>"
  Bus Selector1/2 -> Mux2/2  "<Y>"
  Bus Selector1/1 -> Mux2/1  "<X>"
  Reshape/1 -> Sum/1
  Bus Creator3/1 -> VehSusp/1  "Veh"
  Reshape2/1 -> VehVbody/1  "V"
  Veh/1 -> Bus Selector1/1, Bus Selector2/1, Bus Selector3/1

== system Vehicle14DOFSystemRack/Vehicle 14 DoF model/Vehicle 14 DoF model/Front Suspension/Kinematics and Compliance Independent Suspension/Wheel  Adapter ==
  Wheels : Inport
  Bus Selector : BusSelector  OutputSignals=SuspFrame.Fx,SuspFrame.Fy
  Bus Selector1 : BusSelector  OutputSignals=SuspFrame.Re
  Bus Selector2 : BusSelector  OutputSignals=SuspFrame.Mx,SuspFrame.My,SuspFrame.Mz
  Bus Selector3 : BusSelector  OutputSignals=SuspFrame.z,SuspFrame.zdot
  Matrix Concatenate : Concatenate  NumInputs=3  Mode=Multidimensional array
  Reshape{,1..7} (8 alike) : Reshape  OutputDimensionality=Row vector (2-D)
  WhlFx : Outport  VectorParamsAs1DForOutWhenUnconnected=off
  WhlFy : Outport  Port=2  VectorParamsAs1DForOutWhenUnconnected=off
  z : Outport  Port=3  VectorParamsAs1DForOutWhenUnconnected=off
  zdot : Outport  Port=4  VectorParamsAs1DForOutWhenUnconnected=off
  M : Outport  Port=5  VectorParamsAs1DForOutWhenUnconnected=off
  Re : Outport  Port=6  VectorParamsAs1DForOutWhenUnconnected=off
  wires:
  Reshape/1 -> z/1  "z"
  Matrix Concatenate/1 -> M/1  "M"
  Reshape5/1 -> Matrix Concatenate/3
  Reshape4/1 -> Matrix Concatenate/2
  Reshape3/1 -> Matrix Concatenate/1
  Bus Selector2/3 -> Reshape5/1  "<Mz>"
  Bus Selector2/2 -> Reshape4/1  "<My>"
  Bus Selector2/1 -> Reshape3/1  "<Mx>"
  Reshape1/1 -> Re/1  "Re"
  Bus Selector1/1 -> Reshape1/1  "<Re>"
  Reshape2/1 -> zdot/1  "zdot"
  Bus Selector3/2 -> Reshape2/1  "<zdot>"
  Wheels/1 -> Bus Selector/1, Bus Selector3/1, Bus Selector2/1, Bus Selector1/1
  Bus Selector3/1 -> Reshape/1  "<z>"
  Bus Selector/2 -> Reshape7/1  "<Fy>"
  Bus Selector/1 -> Reshape6/1  "<Fx>"
  Reshape6/1 -> WhlFx/1
  Reshape7/1 -> WhlFy/1

== system Vehicle14DOFSystemRack/Vehicle 14 DoF model/Vehicle 14 DoF model/Front Suspension/Susp2Wheel/Veh2Tire ==
  SteerAng : Inport
  SteerCmb : Inport  Port=2
  Fz : Inport  Port=3
  r : Inport  Port=4
  VehVel : Inport  Port=5
  Reshape1 : Reshape
  Reshape2 : Reshape
  Reshape5 : Reshape
  Unary Minus : UnaryMinus
  Wheel Angles : Subsystem
  Wheel to Body Transform : Subsystem
  WhlAng : Outport  Unit=rad  VectorParamsAs1DForOutWhenUnconnected=off
  YawRate : Outport  Port=2  Unit=rad/s  VectorParamsAs1DForOutWhenUnconnected=off
  Vx : Outport  Port=3  Unit=m/s  VectorParamsAs1DForOutWhenUnconnected=off
  Vy : Outport  Port=4  Unit=m/s  VectorParamsAs1DForOutWhenUnconnected=off
  Vz : Outport  Port=5  Unit=m/s  VectorParamsAs1DForOutWhenUnconnected=off
  Fext : Outport  Port=6  Unit=N  VectorParamsAs1DForOutWhenUnconnected=off
  wires:
  SteerCmb/1 -> Wheel Angles/2(SteerCmb)
  Reshape5/1 -> Vz/1
  Reshape2/1 -> Vy/1
  Reshape1/1 -> Vx/1
  Wheel Angles/1("WhlAng ") -> Wheel to Body Transform/2(WheelAngles), WhlAng/1
  Unary Minus/1 -> YawRate/1
  Wheel to Body Transform/3(zdotWheel) -> Reshape5/1  "Vz"
  VehVel/1 -> Wheel to Body Transform/1(VelVeh)
  r/1 -> Unary Minus/1
  SteerAng/1 -> Wheel Angles/1(SteerAng)
  Wheel to Body Transform/2(ydotWheel) -> Reshape2/1  "Vy"
  Wheel to Body Transform/1(xdotWheel) -> Reshape1/1  "Vx"
  Fz/1 -> Fext/1

== system Vehicle14DOFSystemRack/Vehicle 14 DoF model/Vehicle 14 DoF model/Front Suspension/Wheel2Susp/Suspension Routing ==
  Omega : Inport
  Fx : Inport  Port=2
  Fy : Inport  Port=3
  Fz : Inport  Port=4
  <Mx> : Inport  Port=5
  <My> : Inport  Port=6
  <Mz> : Inport  Port=7
  <Re> : Inport  Port=8
  <z> : Inport  Port=9
  <zdot> : Inport  Port=10
  <Kappa> : Inport  Port=11
  <Alpha> : Inport  Port=12
  Veh : Inport  Port=13
  Bus Creator : BusCreator  Inputs=13
  Bus Selector3 : BusSelector  OutputSignals=InertFrm.FrntAxl.Lft.Disp.Z,InertFrm.FrntAxl.Rght.Disp.Z,InertFrm.RearAxl.Lft.Disp.Z,InertFrm.RearAxl.Rght.Disp.Z
  Bus Selector4 : BusSelector  OutputSignals=BdyFrm.FrntAxl.Lft.Disp.z,BdyFrm.FrntAxl.Rght.Disp.z,BdyFrm.RearAxl.Lft.Disp.z,BdyFrm.RearAxl.Rght.Disp.z
  Subtract : Sum  Inputs=--+
  Unary Minus1 : UnaryMinus
  Unary Minus2 : UnaryMinus
  Vector Concatenate3 : Concatenate  NumInputs=4
  Vector Concatenate4 : Concatenate  NumInputs=4
  SuspFrame : Outport  VectorParamsAs1DForOutWhenUnconnected=off
  wires:
  Bus Selector4/3 -> Vector Concatenate4/3  "<z>"
  Bus Selector4/4 -> Vector Concatenate4/4  "<z>"
  Bus Selector3/2 -> Vector Concatenate3/2  "<Z>"
  Bus Selector3/3 -> Vector Concatenate3/3  "<Z>"
  Bus Selector4/2 -> Vector Concatenate4/2  "<z>"
  Vector Concatenate4/1 -> Subtract/2
  Vector Concatenate3/1 -> Subtract/3
  Bus Selector3/1 -> Vector Concatenate3/1  "<Z>"
  Bus Selector4/1 -> Vector Concatenate4/1  "<z>"
  Subtract/1 -> Bus Creator/9  "dz"
  Bus Selector3/4 -> Vector Concatenate3/4  "<Z>"
  Veh/1 -> Bus Selector4/1, Bus Selector3/1
  <Alpha>/1 -> Bus Creator/13
  <My>/1 -> Bus Creator/6  "My"
  <Mx>/1 -> Bus Creator/5  "Mx"
  <Kappa>/1 -> Bus Creator/12
  Fx/1 -> Bus Creator/2  "Fx"
  Omega/1 -> Bus Creator/1  "Omega"
  Fy/1 -> Bus Creator/3  "Fy"
  Bus Creator/1 -> SuspFrame/1
  <z>/1 -> Unary Minus1/1
  Unary Minus2/1 -> Bus Creator/11  "zdot"
  <Mz>/1 -> Bus Creator/7  "Mz"
  <zdot>/1 -> Unary Minus2/1
  Fz/1 -> Bus Creator/4  "Fz"
  Unary Minus1/1 -> Bus Creator/10, Subtract/1  "z"
  <Re>/1 -> Bus Creator/8

== system Vehicle14DOFSystemRack/Vehicle 14 DoF model/Vehicle 14 DoF model/Front Suspension/Wheel2Susp/Wheel to Body Transform ==
  Forces : Inport  PortDimensions=[3,1]  Partition=on  PartitionDimension=2  PartitionWidth=1  PartitionOffset=0
  Moments : Inport  Port=2  PortDimensions=[3,1]  Partition=on  PartitionDimension=2  PartitionWidth=1  PartitionOffset=0
  DCM : Inport  Port=3  Partition=on  PartitionDimension=3  PartitionWidth=1  PartitionOffset=0
  WheelAngles : Inport  Port=4  Partition=on  PartitionDimension=2  PartitionWidth=1  PartitionOffset=0
  Re : Inport  Port=5  Partition=on  PartitionDimension=1  PartitionWidth=1  PartitionOffset=0
  Add : Sum
  Constant : Constant  Value=[pi;0;0]
  Constant1 : Constant  Value=zeros(2,1)
  Cross Product : matrix_library/Cross Product
  Demux1 : Demux  Outputs=3
  Demux2 : Demux  Outputs=3
  Divide1 : Product  Inputs=***  Multiplication=Matrix(*)
  Divide2 : Product  Inputs=**  Multiplication=Matrix(*)
  Divide3 : Product  Inputs=**  Multiplication=Matrix(*)
  For Each : ForEach  DisableCoverage=on
  Mux : Mux  Inputs=2
  Rotation Angles to Direction Cosine Matrix : autolibsharedcommon/Rotation Angles to Direction Cosine Matrix  rotationOrder=ZYX  aMode=aMode
      settings: AttributesFormatString=Rotation Order: %<rotationOrder>
  Rotation Angles to Direction Cosine Matrix1 : autolibsharedcommon/Rotation Angles to Direction Cosine Matrix  rotationOrder=ZYX  aMode=aMode
      settings: AttributesFormatString=Rotation Order: %<rotationOrder>
  Selector : Selector  InputPortWidth=3  IndexOptions=Index vector (dialog)  Indices=[3 2 1]  OutputSizes=1
  Selector1 : Selector  InputPortWidth=3  IndexOptions=Index vector (dialog)  Indices=[3 2 1]  OutputSizes=1
  Transpose : Math  Operator=transpose
  Transpose1 : Math  Operator=transpose
  Fx : Outport  ConcatenationDimension=1  VectorParamsAs1DForOutWhenUnconnected=off
  Fy : Outport  Port=2  ConcatenationDimension=1  VectorParamsAs1DForOutWhenUnconnected=off
  Fz : Outport  Port=3  ConcatenationDimension=1  VectorParamsAs1DForOutWhenUnconnected=off
  Mx : Outport  Port=4  ConcatenationDimension=1  VectorParamsAs1DForOutWhenUnconnected=off
  My : Outport  Port=5  ConcatenationDimension=1  VectorParamsAs1DForOutWhenUnconnected=off
  Mz : Outport  Port=6  ConcatenationDimension=1  VectorParamsAs1DForOutWhenUnconnected=off
  wires:
  Demux1/1 -> Fx/1
  Demux1/2 -> Fy/1
  Demux1/3 -> Fz/1
  Rotation Angles to Direction Cosine Matrix/1 -> Transpose/1
  Forces/1 -> Divide2/2, Cross Product/2
  WheelAngles/1 -> Selector/1
  Selector/1 -> Rotation Angles to Direction Cosine Matrix/1
  Rotation Angles to Direction Cosine Matrix1/1 -> Divide1/3
  Selector1/1 -> Rotation Angles to Direction Cosine Matrix1/1
  Constant/1 -> Selector1/1
  Transpose/1 -> Divide1/2
  DCM/1 -> Transpose1/1
  Transpose1/1 -> Divide1/1
  Divide2/1 -> Demux1/1
  Divide3/1 -> Demux2/1
  Divide1/1 -> Divide3/1, Divide2/1
  Moments/1 -> Add/2
  Demux2/3 -> Mz/1
  Demux2/2 -> My/1
  Demux2/1 -> Mx/1
  Add/1 -> Divide3/2
  Cross Product/1 -> Add/1
  Mux/1 -> Cross Product/1
  Re/1 -> Mux/2
  Constant1/1 -> Mux/1

== system Vehicle14DOFSystemRack/Vehicle 14 DoF model/Vehicle 14 DoF model/Front Suspension/Wheel2SuspFrntOnly/Suspension Routing ==
  Omega : Inport
  Fx : Inport  Port=2
  Fy : Inport  Port=3
  Fz : Inport  Port=4
  <Mx> : Inport  Port=5
  <My> : Inport  Port=6
  <Mz> : Inport  Port=7
  <Re> : Inport  Port=8
  <z> : Inport  Port=9
  <zdot> : Inport  Port=10
  <Kappa> : Inport  Port=11
  <Alpha> : Inport  Port=12
  Veh : Inport  Port=13
  Bus Creator : BusCreator  Inputs=13
  Bus Selector3 : BusSelector  OutputSignals=InertFrm.FrntAxl.Lft.Disp.Z,InertFrm.FrntAxl.Rght.Disp.Z
  Bus Selector4 : BusSelector  OutputSignals=BdyFrm.FrntAxl.Lft.Disp.z,BdyFrm.FrntAxl.Rght.Disp.z
  Subtract : Sum  Inputs=--+
  Unary Minus1 : UnaryMinus
  Unary Minus2 : UnaryMinus
  Vector Concatenate3 : Concatenate
  Vector Concatenate4 : Concatenate
  SuspFrame : Outport  VectorParamsAs1DForOutWhenUnconnected=off
  wires:
  Bus Selector3/2 -> Vector Concatenate3/2  "<Z>"
  Bus Selector4/2 -> Vector Concatenate4/2  "<z>"
  Vector Concatenate4/1 -> Subtract/2
  Vector Concatenate3/1 -> Subtract/3
  Bus Selector3/1 -> Vector Concatenate3/1  "<Z>"
  Bus Selector4/1 -> Vector Concatenate4/1  "<z>"
  Subtract/1 -> Bus Creator/9  "dz"
  Veh/1 -> Bus Selector4/1, Bus Selector3/1
  <Alpha>/1 -> Bus Creator/13
  <My>/1 -> Bus Creator/6  "My"
  <Mx>/1 -> Bus Creator/5  "Mx"
  <Kappa>/1 -> Bus Creator/12
  Fx/1 -> Bus Creator/2  "Fx"
  Omega/1 -> Bus Creator/1  "Omega"
  Fy/1 -> Bus Creator/3  "Fy"
  Bus Creator/1 -> SuspFrame/1
  <z>/1 -> Unary Minus1/1
  Unary Minus2/1 -> Bus Creator/11  "zdot"
  <Mz>/1 -> Bus Creator/7  "Mz"
  <zdot>/1 -> Unary Minus2/1
  Fz/1 -> Bus Creator/4  "Fz"
  Unary Minus1/1 -> Bus Creator/10, Subtract/1  "z"
  <Re>/1 -> Bus Creator/8

== system Vehicle14DOFSystemRack/Vehicle 14 DoF model/Vehicle 14 DoF model/Front Suspension/Wheel2SuspFrntOnly/Wheel to Body Transform ==
  Forces : Inport  PortDimensions=[3,1]  Partition=on  PartitionDimension=2  PartitionWidth=1  PartitionOffset=0
  Moments : Inport  Port=2  PortDimensions=[3,1]  Partition=on  PartitionDimension=2  PartitionWidth=1  PartitionOffset=0
  DCM : Inport  Port=3  Partition=on  PartitionDimension=3  PartitionWidth=1  PartitionOffset=0
  WheelAngles : Inport  Port=4  Partition=on  PartitionDimension=2  PartitionWidth=1  PartitionOffset=0
  Re : Inport  Port=5  Partition=on  PartitionDimension=1  PartitionWidth=1  PartitionOffset=0
  Add : Sum
  Constant : Constant  Value=[pi;0;0]
  Constant1 : Constant  Value=zeros(2,1)
  Cross Product : matrix_library/Cross Product
  Demux1 : Demux  Outputs=3
  Demux2 : Demux  Outputs=3
  Divide1 : Product  Inputs=***  Multiplication=Matrix(*)
  Divide2 : Product  Inputs=**  Multiplication=Matrix(*)
  Divide3 : Product  Inputs=**  Multiplication=Matrix(*)
  For Each : ForEach  DisableCoverage=on
  Mux : Mux  Inputs=2
  Rotation Angles to Direction Cosine Matrix : autolibsharedcommon/Rotation Angles to Direction Cosine Matrix  rotationOrder=ZYX  aMode=aMode
      settings: AttributesFormatString=Rotation Order: %<rotationOrder>
  Rotation Angles to Direction Cosine Matrix1 : autolibsharedcommon/Rotation Angles to Direction Cosine Matrix  rotationOrder=ZYX  aMode=aMode
      settings: AttributesFormatString=Rotation Order: %<rotationOrder>
  Selector : Selector  InputPortWidth=3  IndexOptions=Index vector (dialog)  Indices=[3 2 1]  OutputSizes=1
  Selector1 : Selector  InputPortWidth=3  IndexOptions=Index vector (dialog)  Indices=[3 2 1]  OutputSizes=1
  Transpose : Math  Operator=transpose
  Transpose1 : Math  Operator=transpose
  Fx : Outport  ConcatenationDimension=1  VectorParamsAs1DForOutWhenUnconnected=off
  Fy : Outport  Port=2  ConcatenationDimension=1  VectorParamsAs1DForOutWhenUnconnected=off
  Fz : Outport  Port=3  ConcatenationDimension=1  VectorParamsAs1DForOutWhenUnconnected=off
  Mx : Outport  Port=4  ConcatenationDimension=1  VectorParamsAs1DForOutWhenUnconnected=off
  My : Outport  Port=5  ConcatenationDimension=1  VectorParamsAs1DForOutWhenUnconnected=off
  Mz : Outport  Port=6  ConcatenationDimension=1  VectorParamsAs1DForOutWhenUnconnected=off
  wires:
  Demux1/1 -> Fx/1
  Demux1/2 -> Fy/1
  Demux1/3 -> Fz/1
  Rotation Angles to Direction Cosine Matrix/1 -> Transpose/1
  Forces/1 -> Divide2/2, Cross Product/2
  WheelAngles/1 -> Selector/1
  Selector/1 -> Rotation Angles to Direction Cosine Matrix/1
  Rotation Angles to Direction Cosine Matrix1/1 -> Divide1/3
  Selector1/1 -> Rotation Angles to Direction Cosine Matrix1/1
  Constant/1 -> Selector1/1
  Transpose/1 -> Divide1/2
  DCM/1 -> Transpose1/1
  Transpose1/1 -> Divide1/1
  Divide2/1 -> Demux1/1
  Divide3/1 -> Demux2/1
  Divide1/1 -> Divide3/1, Divide2/1
  Moments/1 -> Add/2
  Demux2/3 -> Mz/1
  Demux2/2 -> My/1
  Demux2/1 -> Mx/1
  Add/1 -> Divide3/2
  Cross Product/1 -> Add/1
  Mux/1 -> Cross Product/1
  Re/1 -> Mux/2
  Constant1/1 -> Mux/1

== system Vehicle14DOFSystemRack/Vehicle 14 DoF model/Vehicle 14 DoF model/Front Wheels/Subsystem/scale factors with friction ==
  lamda_mu_x : Inport
  lamda_mu_y : Inport  Port=2
  0 : Constant  Value=[zeros(1,numWheels)]  VectorParams1D=off
  1 : Constant  Value=[zeros(2,numWheels)]+1  VectorParams1D=off
  2 : Constant  Value=[zeros(1,numWheels)]+1  VectorParams1D=off
  Reshape : Reshape  OutputDimensionality=Row vector (2-D)  OutputDimensions=[1,numWheels]
  Reshape1 : Reshape  OutputDimensionality=Row vector (2-D)  OutputDimensions=[1,numWheels]
  Signal Specification3 : SignalSpecification  Unit=1
  Vector Concatenate : Concatenate  NumInputs=9  Mode=Multidimensional array
  ones : Constant  Value=[ones(6,numWheels)]  VectorParams1D=off
  ones1 : Constant  Value=[ones(9,numWheels)]  VectorParams1D=off
  ones2 : Constant  Value=ones(1,numWheels)  VectorParams1D=off
  ones3 : Constant  Value=[ones(5,numWheels)]  VectorParams1D=off
  lambdas : Outport  Unit=1  VectorParamsAs1DForOutWhenUnconnected=off
  wires:
  ones3/1 -> Vector Concatenate/7
  2/1 -> Vector Concatenate/6  "lam_Vy"
  ones1/1 -> Vector Concatenate/5
  1/1 -> Vector Concatenate/8  "lam_Vykappa"
  Signal Specification3/1 -> lambdas/1
  Reshape/1 -> Vector Concatenate/2
  Reshape1/1 -> Vector Concatenate/3
  0/1 -> Vector Concatenate/4  "lamda_mu_V"
  ones/1 -> Vector Concatenate/9
  Vector Concatenate/1 -> Signal Specification3/1
  ones2/1 -> Vector Concatenate/1  "lambda_Fz0"
  lamda_mu_x/1 -> Reshape/1
  lamda_mu_y/1 -> Reshape1/1

== system Vehicle14DOFSystemRack/Vehicle 14 DoF model/Vehicle 14 DoF model/Rear Suspension/Kinematics and Compliance Independent Suspension/Calculate dynamic track width from lateral wheel center displacement change ==
  dWhlY : Inport
  dWhlZ : Inport  Port=2
  Front Track Calculation : Subsystem
  Gain : Gain  Gain=-1
  Rear Track Calculation : Subsystem
  Sign : Signum  ZeroCross=off
  Vector Concatenate : Concatenate
  w : Outport
  wires:
  Gain/1 -> Sign/1
  Sign/1 -> Front Track Calculation/2(sign), Rear Track Calculation/2(sign)
  Rear Track Calculation/1(w_rear) -> Vector Concatenate/2
  Front Track Calculation/1(w_front) -> Vector Concatenate/1
  Vector Concatenate/1 -> w/1
  dWhlY/1 -> Front Track Calculation/1(dWhlY), Rear Track Calculation/1(dWhlY)
  dWhlZ/1 -> Gain/1
